simulink model "sl_robot_sincrono_control_linea"  (R2016b)
settings: Solver=VariableStepAuto  StartTime=0.0  StopTime=tsim  RelTol=1e-3
values from neighbouring files (symbols this model uses):
  a = in(1)    [control_linea.m]    (also in pruebas_control_P2.m = -1)
  b = in(2)    [control_linea.m]    (also in pruebas_control_P2.m = 1)
  c = in(3)    [control_linea.m]    (also in pruebas_control_P2.m = -1)
  omega_sat = [-0.2618 0.2618]    [prueba_persecucionPURA.m]    (also in pruebas_MCD.m; pruebas_MCI.m; pruebas_control.m; pruebas_control_P2.m)
  pos_init = [0;0;0]    [prueba_persecucionPURA.m]    (also in pruebas_MCD.m; pruebas_MCI.m; pruebas_control.m; pruebas_control_P2.m)
  tetha_d_sat = [-0.75 0.75]    [prueba_persecucionPURA.m]    (also in pruebas_MCD.m; pruebas_MCI.m; pruebas_control.m; pruebas_control_P2.m)
settings Model: Creator=marrcogrova  LastModifiedBy=marrcogrova

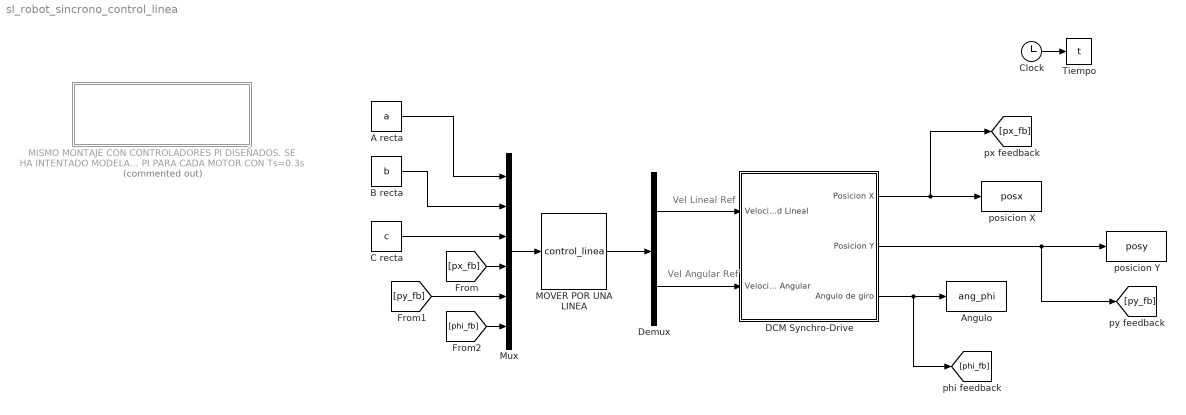
== system sl_robot_sincrono_control_linea ==
  note: Vel Lineal Ref
  note: Vel Angular Ref
  A recta : Constant  Value=a
  Angulo : ToWorkspace  VariableName=ang_phi  SampleTime=-1
  B recta : Constant  Value=b
  C recta : Constant  Value=c
  Clock : Clock
  DCM Synchro-Drive : Subsystem
  Demux : Demux  Outputs=2
  MISMO MONTAJE CON CONTROLADORES PI DISEÑADOS. SE HA INTENTADO MODELAR LOS MOTORES Y DISEÑAR UN PI PARA CADA MOTOR CON Ts=0.3s : Subsystem  Commented=on
  MOVER POR UNA LINEA : MATLABFcn  MATLABFcn=control_linea  OutputDimensions=2
  Mux : Mux  Inputs=6
  Tiempo : ToWorkspace  VariableName=t  SampleTime=-1
  posicion X : ToWorkspace  VariableName=posx  SampleTime=-1
  posicion Y : ToWorkspace  VariableName=posy  SampleTime=-1
  wires:
  Clock/1 -> Tiempo/1
  DCM Synchro-Drive/2(Posicion Y) -> [py_fb], posicion Y/1
  MOVER POR UNA LINEA/1 -> Demux/1
  Mux/1 -> MOVER POR UNA LINEA/1
  A recta/1 -> Mux/1
  B recta/1 -> Mux/2
  DCM Synchro-Drive/1(Posicion X) -> [px_fb], posicion X/1
  DCM Synchro-Drive/3(Angulo de giro) -> [phi_fb], Angulo/1
  [phi_fb] -> Mux/6
  [py_fb] -> Mux/5
  [px_fb] -> Mux/4
  C recta/1 -> Mux/3
  Demux/1 -> DCM Synchro-Drive/1(Velocidad Lineal)
  Demux/2 -> DCM Synchro-Drive/2(Velocidad Angular)

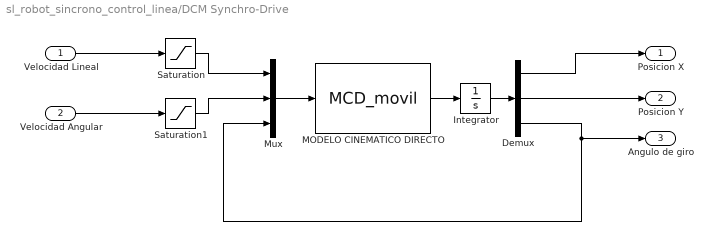
== system sl_robot_sincrono_control_linea/DCM Synchro-Drive ==
  Velocidad Lineal : Inport
  Velocidad Angular : Inport  Port=2
  Demux : Demux  Outputs=3
  Integrator : Integrator  InitialCondition=pos_init
  MODELO CINEMATICO DIRECTO : MATLABFcn  MATLABFcn=MCD_movil  OutputDimensions=3
  Mux : Mux  Inputs=3
  Saturation : Saturate  UpperLimit=tetha_d_sat(2)  LowerLimit=tetha_d_sat(1)
  Saturation1 : Saturate  UpperLimit=omega_sat(2)  LowerLimit=omega_sat(1)
  Posicion X : Outport
  Posicion Y : Outport  Port=2
  Angulo de giro : Outport  Port=3
  wires:
  Integrator/1 -> Demux/1
  Demux/3 -> Angulo de giro/1, Mux/3
  Demux/1 -> Posicion X/1
  Demux/2 -> Posicion Y/1
  Mux/1 -> MODELO CINEMATICO DIRECTO/1
  MODELO CINEMATICO DIRECTO/1 -> Integrator/1
  Velocidad Lineal/1 -> Saturation/1
  Saturation/1 -> Mux/1
  Saturation1/1 -> Mux/2
  Velocidad Angular/1 -> Saturation1/1

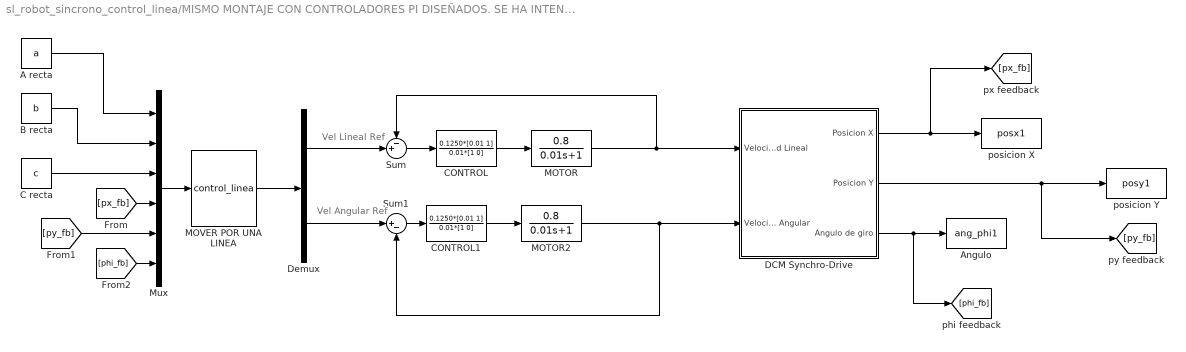
== system sl_robot_sincrono_control_linea/MISMO MONTAJE CON CONTROLADORES PI DISEÑADOS. SE HA INTENTADO MODELAR LOS MOTORES Y DISEÑAR UN PI PARA CADA MOTOR CON Ts=0.3s ==
  note: Vel Lineal Ref
  note: Vel Angular Ref
  A recta : Constant  Value=a
  Angulo : ToWorkspace  VariableName=ang_phi1  SampleTime=-1
  B recta : Constant  Value=b
  C recta : Constant  Value=c
  CONTROL : TransferFcn  Numerator=0.1250*[0.01 1]  Denominator=0.01*[1 0]
  CONTROL1 : TransferFcn  Numerator=0.1250*[0.01 1]  Denominator=0.01*[1 0]
  DCM Synchro-Drive : Subsystem
  Demux : Demux  Outputs=2
  MOTOR : TransferFcn  Numerator=0.8  Denominator=[0.01 1]
  MOTOR2 : TransferFcn  Numerator=0.8  Denominator=[0.01 1]
  MOVER POR UNA LINEA : MATLABFcn  MATLABFcn=control_linea  OutputDimensions=2
  Mux : Mux  Inputs=6
  Sum : Sum  Inputs=-+|
  Sum1 : Sum  Inputs=|+-
  posicion X : ToWorkspace  VariableName=posx1  SampleTime=-1
  posicion Y : ToWorkspace  VariableName=posy1  SampleTime=-1
  wires:
  DCM Synchro-Drive/2(Posicion Y) -> [py_fb], posicion Y/1
  MOVER POR UNA LINEA/1 -> Demux/1
  Mux/1 -> MOVER POR UNA LINEA/1
  A recta/1 -> Mux/1
  B recta/1 -> Mux/2
  DCM Synchro-Drive/1(Posicion X) -> [px_fb], posicion X/1
  DCM Synchro-Drive/3(Angulo de giro) -> [phi_fb], Angulo/1
  [phi_fb] -> Mux/6
  [py_fb] -> Mux/5
  [px_fb] -> Mux/4
  C recta/1 -> Mux/3
  Demux/1 -> Sum/2
  Sum/1 -> CONTROL/1
  Demux/2 -> Sum1/1
  Sum1/1 -> CONTROL1/1
  MOTOR2/1 -> DCM Synchro-Drive/2(Velocidad Angular), Sum1/2
  MOTOR/1 -> DCM Synchro-Drive/1(Velocidad Lineal), Sum/1
  CONTROL/1 -> MOTOR/1
  CONTROL1/1 -> MOTOR2/1

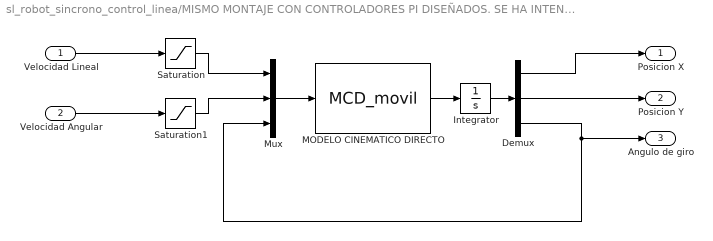
== system sl_robot_sincrono_control_linea/MISMO MONTAJE CON CONTROLADORES PI DISEÑADOS. SE HA INTENTADO MODELAR LOS MOTORES Y DISEÑAR UN PI PARA CADA MOTOR CON Ts=0.3s/DCM Synchro-Drive ==
  Velocidad Lineal : Inport
  Velocidad Angular : Inport  Port=2
  Demux : Demux  Outputs=3
  Integrator : Integrator  InitialCondition=pos_init
  MODELO CINEMATICO DIRECTO : MATLABFcn  MATLABFcn=MCD_movil  OutputDimensions=3
  Mux : Mux  Inputs=3
  Saturation : Saturate  UpperLimit=tetha_d_sat(2)  LowerLimit=tetha_d_sat(1)
  Saturation1 : Saturate  UpperLimit=omega_sat(2)  LowerLimit=omega_sat(1)
  Posicion X : Outport
  Posicion Y : Outport  Port=2
  Angulo de giro : Outport  Port=3
  wires:
  Integrator/1 -> Demux/1
  Demux/3 -> Angulo de giro/1, Mux/3
  Demux/1 -> Posicion X/1
  Demux/2 -> Posicion Y/1
  Mux/1 -> MODELO CINEMATICO DIRECTO/1
  MODELO CINEMATICO DIRECTO/1 -> Integrator/1
  Velocidad Lineal/1 -> Saturation/1
  Saturation/1 -> Mux/1
  Saturation1/1 -> Mux/2
  Velocidad Angular/1 -> Saturation1/1
